simulink model "PI_Controller"  (R2025b)
settings: Solver=VariableStepAuto  StartTime=0.0  StopTime=10.0  RelTol=1e-3
model workspace (MAT data in the model file):
  Ts = 0.01
  ki = 7.33
  kp = 9.39

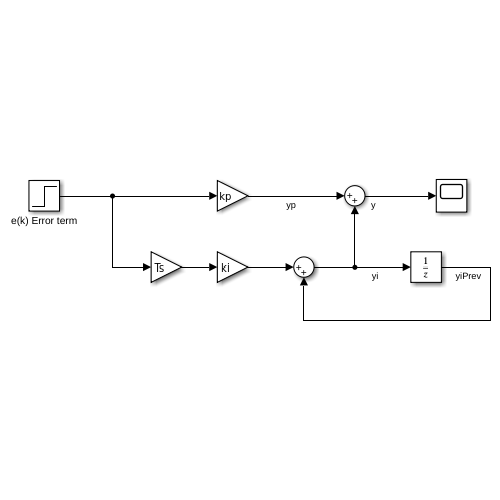
[thumbnail: Simulink's stored preview of the top-level diagram]
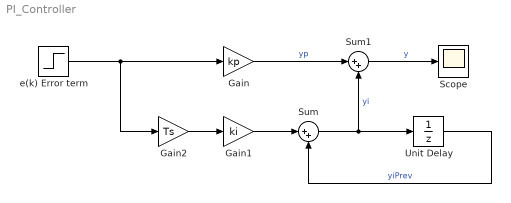
== system PI_Controller ==
  Gain : Gain  Gain=kp
  Gain1 : Gain  Gain=ki
  Gain2 : Gain  Gain=Ts
  Scope : Scope
      settings: ActiveDisplayYMinimum=-9.4291625000001726  ActiveDisplayYMaximum=84.86246250000157
  Sum : Sum  Inputs=|++
  Sum1 : Sum  Inputs=|++
  Unit Delay : UnitDelay  SampleTime=Ts  HasFrameUpgradeWarning=on
  e(k) Error term : Step  SampleTime=0
  wires:
  Unit Delay/1 -> Sum/2  "yiPrev"
  Sum/1 -> Unit Delay/1, Sum1/2  "yi"
  e(k) Error term/1 -> Gain2/1, Gain/1
  Gain2/1 -> Gain1/1
  Gain/1 -> Sum1/1  "yp"
  Gain1/1 -> Sum/1
  Sum1/1 -> Scope/1  "y"
